simulink model "ieee80211n"  (Simulink 6.0)
settings: Solver=VariableStepDiscrete  StartTime=0.0  StopTime=inf  RelTol=1e-3
PreLoadFcn:
  | load IEEE80211n_init;
values from neighbouring files (symbols this model uses):
  params =     [IEEE80211n_init.mat]    (also in IEEE80211n_settings.m = p)
undefined symbols (not defined in the file or in its folder): magnitude
libraries: commblkintrlv2 x196, dspsigops x143, simulink x136, commdigbbndam2 x98, dspmtrx3 x96, dspsigattribs x69, dspstat3 x38, commutil2 x32, commsequence2 x26, commcnvcod2 x10, dspindex x9, dspmlti3 x8
(part 4 of 12)

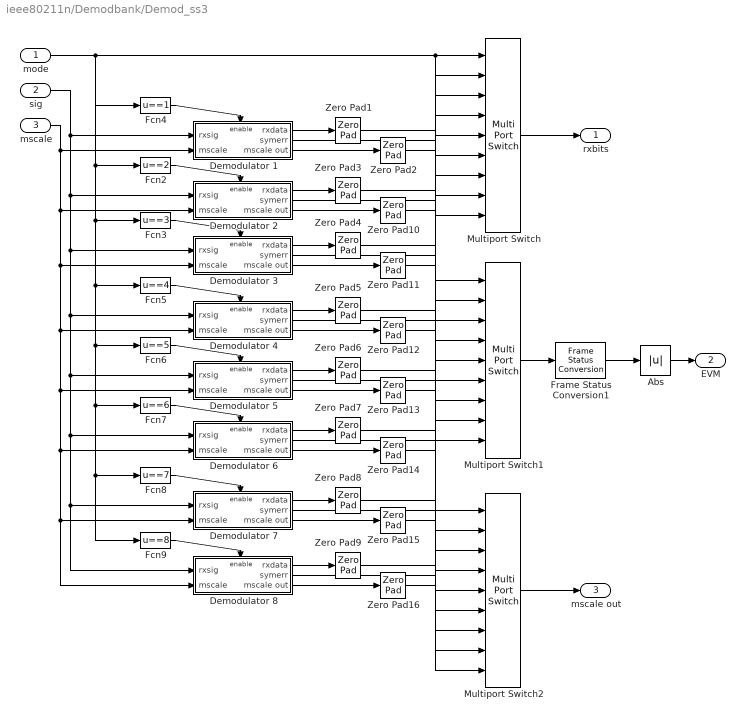
== system ieee80211n/Demodbank/Demod_ss3 ==
  mode : Inport  Port=1  LatchInput=off
  sig : Inport  Port=2  LatchInput=off
  mscale : Inport  Port=3  LatchInput=off
  Abs : Abs  SaturateOnIntegerOverflow=on
  Demodulator 1 : Subsystem  AncestorBlock=IEEE80211a_lib/Demodulator  TreatAsAtomicUnit=on  mask(QAM Demodulator-Decoder.){numSymbols=832, modulation=BPSK, code=1/2, trellisStructure=poly2trellis(7, [171 133]), punctureVector=[1], vtbd=128}
      mask prompts: numSymbols "Number of symbols per frame:"; trellisStructure "Trellis:"; punctureVector "Puncture vector:"; vtbd "Viterbi trace back depth:"
      mask help: Demodulator has option to zero-pad output, so that a bank of different modulators can share the same output frame size.
      mask init:
      | % number of bits per symbol
      | switch modulation
      | 	case 'BPSK', Nb1 = 1;
      | 	case 'QPSK', Nb1 = 2;
      | 	case '16-QAM', Nb1 = 4;
      | 	case '64-QAM', Nb1 = 6;
      | end
      | 
      | modOrder = 2.^Nb1;
      | Nb = numSymbols * Nb1; % tx bits per block
      | codeRate = str2num(strvcat(code)).';
      | bitsPerBlock = Nb .* codeRate;
      | s=max([Nb1/2 1]);
      | 
      | % interleaver
      | interleaverRows = 13;
      | if rem(Nb, interleaverRows)
      | 	error('Number of transmitted bits per block must be multiple of 16.')
      | end
      | interleaverCols = Nb / interleaverRows;
      | interleaverElements = [...
      |             s*floor( [0:Nb-1]/s ) + ...
      |             mod( ([0:Nb-1] + Nb - floor( interleaverRows*[0:Nb-1]/Nb ) ), s ) ...
      |             + 1]';
      | 	
      | if 1 %%%%%%%%%%%%%%%%%%%%%%%%
      | % freq rotation interleaver
      | iss = 2;
      | freqRotNum = 1*11;  % 20MHz channel
      | freqRotInterleaverElements = [...
      |             mod([0:Nb-1] - (mod(2*iss, 3) + 3*floor(iss/3)*freqRotNum*Nb1), Nb) ...
      |             + 1]';
      | end   %%%%%%%%%%%%%%%%%%%%%%%%
      mask Display:
      | disp(['Demodulator\n' modulation ' ' code])
      | port_label('input', 1, ' ')
      | port_label('output', 1, ' ')
      | port_label('output', 2, 'err')
  Demodulator 2 : Subsystem  AncestorBlock=IEEE80211a_lib/Demodulator  TreatAsAtomicUnit=on  mask(QAM Demodulator-Decoder.){numSymbols=832, modulation=QPSK, code=1/2, trellisStructure=poly2trellis(7, [171 133]), punctureVector=[1], vtbd=128}
      mask prompts: numSymbols "Number of symbols per frame:"; trellisStructure "Trellis:"; punctureVector "Puncture vector:"; vtbd "Viterbi trace back depth:"
      mask help: Demodulator has option to zero-pad output, so that a bank of different modulators can share the same output frame size.
      mask init: same as ieee80211n/Demodbank/Demod_ss3/Demodulator 1
      mask Display:
      | disp(['Demodulator\n' modulation ' ' code])
      | port_label('input', 1, ' ')
      | port_label('output', 1, ' ')
      | port_label('output', 2, 'err')
  Demodulator 3 : Subsystem  AncestorBlock=IEEE80211a_lib/Demodulator  TreatAsAtomicUnit=on  mask(QAM Demodulator-Decoder.){numSymbols=832, modulation=QPSK, code=3/4, trellisStructure=poly2trellis(7, [171 133]), punctureVector=[1 1 1 0 0 1].', vtbd=128}
      mask prompts: numSymbols "Number of symbols per frame:"; trellisStructure "Trellis:"; punctureVector "Puncture vector:"; vtbd "Viterbi trace back depth:"
      mask help: Demodulator has option to zero-pad output, so that a bank of different modulators can share the same output frame size.
      mask init: same as ieee80211n/Demodbank/Demod_ss3/Demodulator 1
      mask Display:
      | disp(['Demodulator\n' modulation ' ' code])
      | port_label('input', 1, ' ')
      | port_label('output', 1, ' ')
      | port_label('output', 2, 'err')
  Demodulator 4 : Subsystem  AncestorBlock=IEEE80211a_lib/Demodulator  TreatAsAtomicUnit=on  mask(QAM Demodulator-Decoder.){numSymbols=832, modulation=16-QAM, code=1/2, trellisStructure=poly2trellis(7, [171 133]), punctureVector=[1], vtbd=128}
      mask prompts: numSymbols "Number of symbols per frame:"; trellisStructure "Trellis:"; punctureVector "Puncture vector:"; vtbd "Viterbi trace back depth:"
      mask help: Demodulator has option to zero-pad output, so that a bank of different modulators can share the same output frame size.
      mask init: same as ieee80211n/Demodbank/Demod_ss3/Demodulator 1
      mask Display:
      | disp(['Demodulator\n' modulation ' ' code])
      | port_label('input', 1, ' ')
      | port_label('output', 1, ' ')
      | port_label('output', 2, 'err')
  Demodulator 5 : Subsystem  AncestorBlock=IEEE80211a_lib/Demodulator  TreatAsAtomicUnit=on  mask(QAM Demodulator-Decoder.){numSymbols=832, modulation=16-QAM, code=3/4, trellisStructure=poly2trellis(7, [171 133]), punctureVector=[1 1 1 0 0 1].', vtbd=128}
      mask prompts: numSymbols "Number of symbols per frame:"; trellisStructure "Trellis:"; punctureVector "Puncture vector:"; vtbd "Viterbi trace back depth:"
      mask help: Demodulator has option to zero-pad output, so that a bank of different modulators can share the same output frame size.
      mask init: same as ieee80211n/Demodbank/Demod_ss3/Demodulator 1
      mask Display:
      | disp(['Demodulator\n' modulation ' ' code])
      | port_label('input', 1, ' ')
      | port_label('output', 1, ' ')
      | port_label('output', 2, 'err')
  Demodulator 6 : Subsystem  AncestorBlock=IEEE80211a_lib/Demodulator  TreatAsAtomicUnit=on  mask(QAM Demodulator-Decoder.){numSymbols=832, modulation=64-QAM, code=2/3, trellisStructure=poly2trellis(7, [133 171]), punctureVector=[1 1 1 0].', vtbd=128}
      mask prompts: numSymbols "Number of symbols per frame:"; trellisStructure "Trellis:"; punctureVector "Puncture vector:"; vtbd "Viterbi trace back depth:"
      mask help: Demodulator has option to zero-pad output, so that a bank of different modulators can share the same output frame size.
      mask init: same as ieee80211n/Demodbank/Demod_ss3/Demodulator 1
      mask Display:
      | disp(['Demodulator\n' modulation ' ' code])
      | port_label('input', 1, ' ')
      | port_label('output', 1, ' ')
      | port_label('output', 2, 'err')
  Demodulator 7 : Subsystem  AncestorBlock=IEEE80211a_lib/Demodulator  TreatAsAtomicUnit=on  mask(QAM Demodulator-Decoder.){numSymbols=832, modulation=64-QAM, code=3/4, trellisStructure=poly2trellis(7, [133 171]), punctureVector=[1 1 1 0 0 1].', vtbd=128}
      mask prompts: numSymbols "Number of symbols per frame:"; trellisStructure "Trellis:"; punctureVector "Puncture vector:"; vtbd "Viterbi trace back depth:"
      mask help: Demodulator has option to zero-pad output, so that a bank of different modulators can share the same output frame size.
      mask init: same as ieee80211n/Demodbank/Demod_ss3/Demodulator 1
      mask Display:
      | disp(['Demodulator\n' modulation ' ' code])
      | port_label('input', 1, ' ')
      | port_label('output', 1, ' ')
      | port_label('output', 2, 'err')
  Demodulator 8 : Subsystem  AncestorBlock=IEEE80211a_lib/Demodulator  TreatAsAtomicUnit=on  mask(QAM Demodulator-Decoder.){numSymbols=832, modulation=64-QAM, code=5/6, trellisStructure=poly2trellis(7, [133 171]), punctureVector=[1 1 1 0 0 1 1 0 0 1].', vtbd=128}
      mask prompts: numSymbols "Number of symbols per frame:"; trellisStructure "Trellis:"; punctureVector "Puncture vector:"; vtbd "Viterbi trace back depth:"
      mask help: Demodulator has option to zero-pad output, so that a bank of different modulators can share the same output frame size.
      mask init: same as ieee80211n/Demodbank/Demod_ss3/Demodulator 1
      mask Display:
      | disp(['Demodulator\n' modulation ' ' code])
      | port_label('input', 1, ' ')
      | port_label('output', 1, ' ')
      | port_label('output', 2, 'err')
  Fcn2 : Fcn  Expr=u==2
  Fcn3 : Fcn  Expr=u==3
  Fcn4 : Fcn  Expr=u==1
  Fcn5 : Fcn  Expr=u==4
  Fcn6 : Fcn  Expr=u==5
  Fcn7 : Fcn  Expr=u==6
  Fcn8 : Fcn  Expr=u==7
  Fcn9 : Fcn  Expr=u==8
  Frame Status Conversion1 : dspsigattribs/Frame Status Conversion  growRefPort=off  outframe=Sample-based
  Multiport Switch : MultiPortSwitch  Inputs=8  SaturateOnIntegerOverflow=on
  Multiport Switch1 : MultiPortSwitch  Inputs=8  SaturateOnIntegerOverflow=on
  Multiport Switch2 : MultiPortSwitch  Inputs=8  SaturateOnIntegerOverflow=on
  Zero Pad{1..16} (16 alike) : dspsigops/Zero Pad  padSigAt=End  zpadAlong=Columns  padNumOutRowsSpecMethod=User-specified  numOutRows=params.maxTxBitsPerBlock  padNumOutColsSpecMethod=User-specified  numOutCols=1  trunc_flag=None
      settings: AttributesFormatString=\n
  rxbits : Outport
  EVM : Outport  Port=2
  mscale out : Outport  Port=3
  wires:
  sig/1 -> Demodulator 1/1(rxsig), Demodulator 3/1(rxsig), Demodulator 6/1(rxsig), Demodulator 7/1(rxsig), Demodulator 8/1(rxsig), Demodulator 5/1(rxsig), Demodulator 4/1(rxsig), Demodulator 2/1(rxsig)
  mode/1 -> Multiport Switch1/1, Multiport Switch/1, Multiport Switch2/1, Fcn4/1, Fcn7/1, Fcn8/1, Fcn9/1, Fcn6/1, Fcn5/1, Fcn3/1, Fcn2/1
  Multiport Switch/1 -> rxbits/1
  Zero Pad1/1 -> Multiport Switch/2
  Demodulator 7/1(rxdata) -> Zero Pad8/1
  Demodulator 6/1(rxdata) -> Zero Pad7/1
  Demodulator 5/1(rxdata) -> Zero Pad6/1
  Demodulator 3/1(rxdata) -> Zero Pad4/1
  Demodulator 4/1(rxdata) -> Zero Pad5/1
  Multiport Switch1/1 -> Frame Status Conversion1/1
  Demodulator 1/2(symerr) -> Multiport Switch1/2
  Demodulator 2/2(symerr) -> Multiport Switch1/3
  Demodulator 4/2(symerr) -> Multiport Switch1/5
  Demodulator 5/2(symerr) -> Multiport Switch1/6
  Demodulator 6/2(symerr) -> Multiport Switch1/7
  Demodulator 7/2(symerr) -> Multiport Switch1/8
  Demodulator 3/2(symerr) -> Multiport Switch1/4
  Zero Pad3/1 -> Multiport Switch/3
  Zero Pad4/1 -> Multiport Switch/4
  Zero Pad5/1 -> Multiport Switch/5
  Zero Pad6/1 -> Multiport Switch/6
  Zero Pad7/1 -> Multiport Switch/7
  Zero Pad8/1 -> Multiport Switch/8
  Fcn4/1 -> Demodulator 1/Enable
  Fcn2/1 -> Demodulator 2/Enable
  Fcn3/1 -> Demodulator 3/Enable
  Fcn5/1 -> Demodulator 4/Enable
  Fcn6/1 -> Demodulator 5/Enable
  Fcn7/1 -> Demodulator 6/Enable
  Fcn8/1 -> Demodulator 7/Enable
  Demodulator 1/1(rxdata) -> Zero Pad1/1
  Demodulator 2/1(rxdata) -> Zero Pad3/1
  Frame Status Conversion1/1 -> Abs/1
  Abs/1 -> EVM/1
  Demodulator 8/1(rxdata) -> Zero Pad9/1
  Demodulator 8/2(symerr) -> Multiport Switch1/9
  Zero Pad9/1 -> Multiport Switch/9
  Fcn9/1 -> Demodulator 8/Enable
  mscale/1 -> Demodulator 1/2(mscale), Demodulator 2/2(mscale), Demodulator 3/2(mscale), Demodulator 4/2(mscale), Demodulator 5/2(mscale), Demodulator 6/2(mscale), Demodulator 7/2(mscale), Demodulator 8/2(mscale)
  Multiport Switch2/1 -> mscale out/1
  Demodulator 1/3(mscale out) -> Zero Pad2/1
  Demodulator 2/3(mscale out) -> Zero Pad10/1
  Demodulator 3/3(mscale out) -> Zero Pad11/1
  Demodulator 4/3(mscale out) -> Zero Pad12/1
  Demodulator 5/3(mscale out) -> Zero Pad13/1
  Demodulator 6/3(mscale out) -> Zero Pad14/1
  Demodulator 7/3(mscale out) -> Zero Pad15/1
  Demodulator 8/3(mscale out) -> Zero Pad16/1
  Zero Pad2/1 -> Multiport Switch2/2
  Zero Pad10/1 -> Multiport Switch2/3
  Zero Pad11/1 -> Multiport Switch2/4
  Zero Pad12/1 -> Multiport Switch2/5
  Zero Pad13/1 -> Multiport Switch2/6
  Zero Pad14/1 -> Multiport Switch2/7
  Zero Pad15/1 -> Multiport Switch2/8
  Zero Pad16/1 -> Multiport Switch2/9

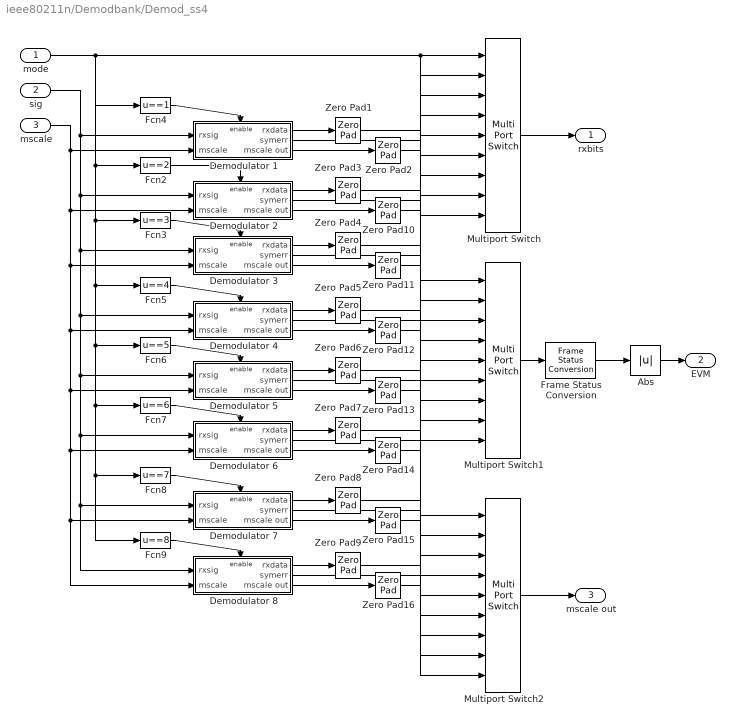
== system ieee80211n/Demodbank/Demod_ss4 ==
  mode : Inport  Port=1  LatchInput=off
  sig : Inport  Port=2  LatchInput=off
  mscale : Inport  Port=3  LatchInput=off
  Abs : Abs  SaturateOnIntegerOverflow=on
  Demodulator 1 : Subsystem  AncestorBlock=IEEE80211a_lib/Demodulator  TreatAsAtomicUnit=on  mask(QAM Demodulator-Decoder.){numSymbols=832, modulation=BPSK, code=1/2, trellisStructure=poly2trellis(7, [171 133]), punctureVector=[1], vtbd=128}
      mask prompts: numSymbols "Number of symbols per frame:"; trellisStructure "Trellis:"; punctureVector "Puncture vector:"; vtbd "Viterbi trace back depth:"
      mask help: Demodulator has option to zero-pad output, so that a bank of different modulators can share the same output frame size.
      mask init:
      | % number of bits per symbol
      | switch modulation
      | 	case 'BPSK', Nb1 = 1;
      | 	case 'QPSK', Nb1 = 2;
      | 	case '16-QAM', Nb1 = 4;
      | 	case '64-QAM', Nb1 = 6;
      | end
      | 
      | modOrder = 2.^Nb1;
      | Nb = numSymbols * Nb1; % tx bits per block
      | codeRate = str2num(strvcat(code)).';
      | bitsPerBlock = Nb .* codeRate;
      | s=max([Nb1/2 1]);
      | 
      | % interleaver
      | interleaverRows = 13;
      | if rem(Nb, interleaverRows)
      | 	error('Number of transmitted bits per block must be multiple of 16.')
      | end
      | interleaverCols = Nb / interleaverRows;
      | interleaverElements = [...
      |             s*floor( [0:Nb-1]/s ) + ...
      |             mod( ([0:Nb-1] + Nb - floor( interleaverRows*[0:Nb-1]/Nb ) ), s ) ...
      |             + 1]';
      | 	
      | if 1 %%%%%%%%%%%%%%%%%%%%%%%%
      | % freq rotation interleaver
      | iss = 3;
      | freqRotNum = 3*11;  % 20MHz channel
      | freqRotInterleaverElements = [...
      |             mod([0:Nb-1] - (mod(2*iss, 3) + 3*floor(iss/3)*freqRotNum*Nb1), Nb) ...
      |             + 1]';
      | end   %%%%%%%%%%%%%%%%%%%%%%%%
      mask Display:
      | disp(['Demodulator\n' modulation ' ' code])
      | port_label('input', 1, ' ')
      | port_label('output', 1, ' ')
      | port_label('output', 2, 'err')
  Demodulator 2 : Subsystem  AncestorBlock=IEEE80211a_lib/Demodulator  TreatAsAtomicUnit=on  mask(QAM Demodulator-Decoder.){numSymbols=832, modulation=QPSK, code=1/2, trellisStructure=poly2trellis(7, [171 133]), punctureVector=[1], vtbd=128}
      mask prompts: numSymbols "Number of symbols per frame:"; trellisStructure "Trellis:"; punctureVector "Puncture vector:"; vtbd "Viterbi trace back depth:"
      mask help: Demodulator has option to zero-pad output, so that a bank of different modulators can share the same output frame size.
      mask init: same as ieee80211n/Demodbank/Demod_ss4/Demodulator 1
      mask Display:
      | disp(['Demodulator\n' modulation ' ' code])
      | port_label('input', 1, ' ')
      | port_label('output', 1, ' ')
      | port_label('output', 2, 'err')
  Demodulator 3 : Subsystem  AncestorBlock=IEEE80211a_lib/Demodulator  TreatAsAtomicUnit=on  mask(QAM Demodulator-Decoder.){numSymbols=832, modulation=QPSK, code=3/4, trellisStructure=poly2trellis(7, [171 133]), punctureVector=[1 1 1 0 0 1].', vtbd=128}
      mask prompts: numSymbols "Number of symbols per frame:"; trellisStructure "Trellis:"; punctureVector "Puncture vector:"; vtbd "Viterbi trace back depth:"
      mask help: Demodulator has option to zero-pad output, so that a bank of different modulators can share the same output frame size.
      mask init: same as ieee80211n/Demodbank/Demod_ss4/Demodulator 1
      mask Display:
      | disp(['Demodulator\n' modulation ' ' code])
      | port_label('input', 1, ' ')
      | port_label('output', 1, ' ')
      | port_label('output', 2, 'err')
  Demodulator 4 : Subsystem  AncestorBlock=IEEE80211a_lib/Demodulator  TreatAsAtomicUnit=on  mask(QAM Demodulator-Decoder.){numSymbols=832, modulation=16-QAM, code=1/2, trellisStructure=poly2trellis(7, [171 133]), punctureVector=[1], vtbd=128}
      mask prompts: numSymbols "Number of symbols per frame:"; trellisStructure "Trellis:"; punctureVector "Puncture vector:"; vtbd "Viterbi trace back depth:"
      mask help: Demodulator has option to zero-pad output, so that a bank of different modulators can share the same output frame size.
      mask init: same as ieee80211n/Demodbank/Demod_ss4/Demodulator 1
      mask Display:
      | disp(['Demodulator\n' modulation ' ' code])
      | port_label('input', 1, ' ')
      | port_label('output', 1, ' ')
      | port_label('output', 2, 'err')
  Demodulator 5 : Subsystem  AncestorBlock=IEEE80211a_lib/Demodulator  TreatAsAtomicUnit=on  mask(QAM Demodulator-Decoder.){numSymbols=832, modulation=16-QAM, code=3/4, trellisStructure=poly2trellis(7, [171 133]), punctureVector=[1 1 1 0 0 1].', vtbd=128}
      mask prompts: numSymbols "Number of symbols per frame:"; trellisStructure "Trellis:"; punctureVector "Puncture vector:"; vtbd "Viterbi trace back depth:"
      mask help: Demodulator has option to zero-pad output, so that a bank of different modulators can share the same output frame size.
      mask init: same as ieee80211n/Demodbank/Demod_ss4/Demodulator 1
      mask Display:
      | disp(['Demodulator\n' modulation ' ' code])
      | port_label('input', 1, ' ')
      | port_label('output', 1, ' ')
      | port_label('output', 2, 'err')
  Demodulator 6 : Subsystem  AncestorBlock=IEEE80211a_lib/Demodulator  TreatAsAtomicUnit=on  mask(QAM Demodulator-Decoder.){numSymbols=832, modulation=64-QAM, code=2/3, trellisStructure=poly2trellis(7, [133 171]), punctureVector=[1 1 1 0].', vtbd=128}
      mask prompts: numSymbols "Number of symbols per frame:"; trellisStructure "Trellis:"; punctureVector "Puncture vector:"; vtbd "Viterbi trace back depth:"
      mask help: Demodulator has option to zero-pad output, so that a bank of different modulators can share the same output frame size.
      mask init: same as ieee80211n/Demodbank/Demod_ss4/Demodulator 1
      mask Display:
      | disp(['Demodulator\n' modulation ' ' code])
      | port_label('input', 1, ' ')
      | port_label('output', 1, ' ')
      | port_label('output', 2, 'err')
  Demodulator 7 : Subsystem  AncestorBlock=IEEE80211a_lib/Demodulator  TreatAsAtomicUnit=on  mask(QAM Demodulator-Decoder.){numSymbols=832, modulation=64-QAM, code=3/4, trellisStructure=poly2trellis(7, [133 171]), punctureVector=[1 1 1 0 0 1].', vtbd=128}
      mask prompts: numSymbols "Number of symbols per frame:"; trellisStructure "Trellis:"; punctureVector "Puncture vector:"; vtbd "Viterbi trace back depth:"
      mask help: Demodulator has option to zero-pad output, so that a bank of different modulators can share the same output frame size.
      mask init: same as ieee80211n/Demodbank/Demod_ss4/Demodulator 1
      mask Display:
      | disp(['Demodulator\n' modulation ' ' code])
      | port_label('input', 1, ' ')
      | port_label('output', 1, ' ')
      | port_label('output', 2, 'err')
  Demodulator 8 : Subsystem  AncestorBlock=IEEE80211a_lib/Demodulator  TreatAsAtomicUnit=on  mask(QAM Demodulator-Decoder.){numSymbols=832, modulation=64-QAM, code=5/6, trellisStructure=poly2trellis(7, [133 171]), punctureVector=[1 1 1 0 0 1 1 0 0 1].', vtbd=128}
      mask prompts: numSymbols "Number of symbols per frame:"; trellisStructure "Trellis:"; punctureVector "Puncture vector:"; vtbd "Viterbi trace back depth:"
      mask help: Demodulator has option to zero-pad output, so that a bank of different modulators can share the same output frame size.
      mask init: same as ieee80211n/Demodbank/Demod_ss4/Demodulator 1
      mask Display:
      | disp(['Demodulator\n' modulation ' ' code])
      | port_label('input', 1, ' ')
      | port_label('output', 1, ' ')
      | port_label('output', 2, 'err')
  Fcn2 : Fcn  Expr=u==2
  Fcn3 : Fcn  Expr=u==3
  Fcn4 : Fcn  Expr=u==1
  Fcn5 : Fcn  Expr=u==4
  Fcn6 : Fcn  Expr=u==5
  Fcn7 : Fcn  Expr=u==6
  Fcn8 : Fcn  Expr=u==7
  Fcn9 : Fcn  Expr=u==8
  Frame Status Conversion : dspsigattribs/Frame Status Conversion  growRefPort=off  outframe=Sample-based
  Multiport Switch : MultiPortSwitch  Inputs=8  SaturateOnIntegerOverflow=on
  Multiport Switch1 : MultiPortSwitch  Inputs=8  SaturateOnIntegerOverflow=on
  Multiport Switch2 : MultiPortSwitch  Inputs=8  SaturateOnIntegerOverflow=on
  Zero Pad{1..16} (16 alike) : dspsigops/Zero Pad  padSigAt=End  zpadAlong=Columns  padNumOutRowsSpecMethod=User-specified  numOutRows=params.maxTxBitsPerBlock  padNumOutColsSpecMethod=User-specified  numOutCols=1  trunc_flag=None
      settings: AttributesFormatString=\n
  rxbits : Outport
  EVM : Outport  Port=2
  mscale out : Outport  Port=3
  wires:
  sig/1 -> Demodulator 1/1(rxsig), Demodulator 3/1(rxsig), Demodulator 6/1(rxsig), Demodulator 7/1(rxsig), Demodulator 8/1(rxsig), Demodulator 5/1(rxsig), Demodulator 4/1(rxsig), Demodulator 2/1(rxsig)
  mode/1 -> Multiport Switch1/1, Multiport Switch/1, Multiport Switch2/1, Fcn4/1, Fcn7/1, Fcn8/1, Fcn9/1, Fcn6/1, Fcn5/1, Fcn3/1, Fcn2/1
  Multiport Switch/1 -> rxbits/1
  Zero Pad1/1 -> Multiport Switch/2
  Demodulator 7/1(rxdata) -> Zero Pad8/1
  Demodulator 6/1(rxdata) -> Zero Pad7/1
  Demodulator 5/1(rxdata) -> Zero Pad6/1
  Demodulator 3/1(rxdata) -> Zero Pad4/1
  Demodulator 4/1(rxdata) -> Zero Pad5/1
  Multiport Switch1/1 -> Frame Status Conversion/1
  Demodulator 1/2(symerr) -> Multiport Switch1/2
  Demodulator 2/2(symerr) -> Multiport Switch1/3
  Demodulator 4/2(symerr) -> Multiport Switch1/5
  Demodulator 5/2(symerr) -> Multiport Switch1/6
  Demodulator 6/2(symerr) -> Multiport Switch1/7
  Demodulator 7/2(symerr) -> Multiport Switch1/8
  Demodulator 3/2(symerr) -> Multiport Switch1/4
  Zero Pad3/1 -> Multiport Switch/3
  Zero Pad4/1 -> Multiport Switch/4
  Zero Pad5/1 -> Multiport Switch/5
  Zero Pad6/1 -> Multiport Switch/6
  Zero Pad7/1 -> Multiport Switch/7
  Zero Pad8/1 -> Multiport Switch/8
  Fcn4/1 -> Demodulator 1/Enable
  Fcn2/1 -> Demodulator 2/Enable
  Fcn3/1 -> Demodulator 3/Enable
  Fcn5/1 -> Demodulator 4/Enable
  Fcn6/1 -> Demodulator 5/Enable
  Fcn7/1 -> Demodulator 6/Enable
  Fcn8/1 -> Demodulator 7/Enable
  Demodulator 1/1(rxdata) -> Zero Pad1/1
  Demodulator 2/1(rxdata) -> Zero Pad3/1
  Frame Status Conversion/1 -> Abs/1
  Abs/1 -> EVM/1
  Demodulator 8/1(rxdata) -> Zero Pad9/1
  Demodulator 8/2(symerr) -> Multiport Switch1/9
  Zero Pad9/1 -> Multiport Switch/9
  Fcn9/1 -> Demodulator 8/Enable
  mscale/1 -> Demodulator 1/2(mscale), Demodulator 2/2(mscale), Demodulator 3/2(mscale), Demodulator 4/2(mscale), Demodulator 5/2(mscale), Demodulator 6/2(mscale), Demodulator 7/2(mscale), Demodulator 8/2(mscale)
  Multiport Switch2/1 -> mscale out/1
  Demodulator 1/3(mscale out) -> Zero Pad2/1
  Demodulator 2/3(mscale out) -> Zero Pad10/1
  Demodulator 3/3(mscale out) -> Zero Pad11/1
  Demodulator 4/3(mscale out) -> Zero Pad12/1
  Demodulator 5/3(mscale out) -> Zero Pad13/1
  Demodulator 6/3(mscale out) -> Zero Pad14/1
  Demodulator 7/3(mscale out) -> Zero Pad15/1
  Demodulator 8/3(mscale out) -> Zero Pad16/1
  Zero Pad2/1 -> Multiport Switch2/2
  Zero Pad10/1 -> Multiport Switch2/3
  Zero Pad11/1 -> Multiport Switch2/4
  Zero Pad12/1 -> Multiport Switch2/5
  Zero Pad13/1 -> Multiport Switch2/6
  Zero Pad14/1 -> Multiport Switch2/7
  Zero Pad15/1 -> Multiport Switch2/8
  Zero Pad16/1 -> Multiport Switch2/9

== system ieee80211n/DocBlock/EmptySubsystem ==

== system ieee80211n/MATLAB graphics/Transform data ==
  in : Inport  Port=1  LatchInput=off
  Complex to Real-Imag : ComplexToRealImag
  Concatenate : simulink/Math Operations/Matrix Concatenation  numInports=2  catMethod=Horizontal
  Frame Status Conversion1 : dspsigattribs/Frame Status Conversion  growRefPort=off  outframe=Sample-based
  out : Outport
  wires:
  Frame Status Conversion1/1 -> out/1
  in/1 -> Complex to Real-Imag/1
  Complex to Real-Imag/1 -> Concatenate/1
  Complex to Real-Imag/2 -> Concatenate/2
  Concatenate/1 -> Frame Status Conversion1/1

== system ieee80211n/MATLAB graphics/append1 ==
  in : Inport  Port=1  LatchInput=off
  Matrix Concatenation1 : simulink/Math Operations/Matrix Concatenation  numInports=2  catMethod=Vertical
  Reshape : simulink/Math Operations/Reshape  OutputDimensionality=Column vector  OutputDimensions=[1,1]
  Transpose : dspmtrx3/Transpose  Hermitian=off  overflowFlag=on
      settings: AttributesFormatString=\n
  Width : Width
  out : Outport
  wires:
  in/1 -> Width/1, Reshape/1
  Width/1 -> Transpose/1
  Reshape/1 -> Matrix Concatenation1/2
  Transpose/1 -> Matrix Concatenation1/1
  Matrix Concatenation1/1 -> out/1

== system ieee80211n/MATLAB graphics/append2 ==
  in : Inport  Port=1  LatchInput=off
  Matrix Concatenation1 : simulink/Math Operations/Matrix Concatenation  numInports=2  catMethod=Vertical
  Reshape : simulink/Math Operations/Reshape  OutputDimensionality=Column vector  OutputDimensions=[1,1]
  Transpose : dspmtrx3/Transpose  Hermitian=off  overflowFlag=on
      settings: AttributesFormatString=\n
  Width : Width
  out : Outport
  wires:
  Matrix Concatenation1/1 -> out/1
  Transpose/1 -> Matrix Concatenation1/1
  Reshape/1 -> Matrix Concatenation1/2
  Width/1 -> Transpose/1
  in/1 -> Reshape/1, Width/1

== system ieee80211n/MATLAB graphics/append3 ==
  in : Inport  Port=1  LatchInput=off
  Matrix Concatenation1 : simulink/Math Operations/Matrix Concatenation  numInports=2  catMethod=Vertical
  Reshape : simulink/Math Operations/Reshape  OutputDimensionality=Column vector  OutputDimensions=[1,1]
  Transpose : dspmtrx3/Transpose  Hermitian=off  overflowFlag=on
      settings: AttributesFormatString=\n
  Width : Width
  out : Outport
  wires:
  Matrix Concatenation1/1 -> out/1
  Transpose/1 -> Matrix Concatenation1/1
  Reshape/1 -> Matrix Concatenation1/2
  Width/1 -> Transpose/1
  in/1 -> Reshape/1, Width/1

== system ieee80211n/MATLAB graphics/append5 ==
  in : Inport  Port=1  LatchInput=off
  Matrix Concatenation1 : simulink/Math Operations/Matrix Concatenation  numInports=2  catMethod=Vertical
  Reshape : simulink/Math Operations/Reshape  OutputDimensionality=Column vector  OutputDimensions=[1,1]
  Transpose : dspmtrx3/Transpose  Hermitian=off  overflowFlag=on
      settings: AttributesFormatString=\n
  Width : Width
  out : Outport
  wires:
  Matrix Concatenation1/1 -> out/1
  Transpose/1 -> Matrix Concatenation1/1
  Reshape/1 -> Matrix Concatenation1/2
  Width/1 -> Transpose/1
  in/1 -> Reshape/1, Width/1

== system ieee80211n/MATLAB graphics/append6 ==
  in : Inport  Port=1  LatchInput=off
  Matrix Concatenation1 : simulink/Math Operations/Matrix Concatenation  numInports=2  catMethod=Vertical
  Reshape : simulink/Math Operations/Reshape  OutputDimensionality=Column vector  OutputDimensions=[1,1]
  Transpose : dspmtrx3/Transpose  Hermitian=off  overflowFlag=on
      settings: AttributesFormatString=\n
  Width : Width
  out : Outport
  wires:
  Matrix Concatenation1/1 -> out/1
  Transpose/1 -> Matrix Concatenation1/1
  Reshape/1 -> Matrix Concatenation1/2
  Width/1 -> Transpose/1
  in/1 -> Reshape/1, Width/1

== system ieee80211n/MATLAB graphics/append7 ==
  in : Inport  Port=1  LatchInput=off
  Matrix Concatenation1 : simulink/Math Operations/Matrix Concatenation  numInports=2  catMethod=Vertical
  Reshape : simulink/Math Operations/Reshape  OutputDimensionality=Column vector  OutputDimensions=[1,1]
  Transpose : dspmtrx3/Transpose  Hermitian=off  overflowFlag=on
      settings: AttributesFormatString=\n
  Width : Width
  out : Outport
  wires:
  Matrix Concatenation1/1 -> out/1
  Transpose/1 -> Matrix Concatenation1/1
  Reshape/1 -> Matrix Concatenation1/2
  Width/1 -> Transpose/1
  in/1 -> Reshape/1, Width/1

== system ieee80211n/MATLAB graphics/append8 ==
  in : Inport  Port=1  LatchInput=off
  Matrix Concatenation1 : simulink/Math Operations/Matrix Concatenation  numInports=2  catMethod=Vertical
  Reshape : simulink/Math Operations/Reshape  OutputDimensionality=Column vector  OutputDimensions=[1,1]
  Transpose : dspmtrx3/Transpose  Hermitian=off  overflowFlag=on
      settings: AttributesFormatString=\n
  Width : Width
  out : Outport
  wires:
  Matrix Concatenation1/1 -> out/1
  Transpose/1 -> Matrix Concatenation1/1
  Reshape/1 -> Matrix Concatenation1/2
  Width/1 -> Transpose/1
  in/1 -> Reshape/1, Width/1

== system ieee80211n/MATLAB graphics/append9 ==
  in : Inport  Port=1  LatchInput=off
  Matrix Concatenation1 : simulink/Math Operations/Matrix Concatenation  numInports=2  catMethod=Vertical
  Reshape : simulink/Math Operations/Reshape  OutputDimensionality=Column vector  OutputDimensions=[1,1]
  Transpose : dspmtrx3/Transpose  Hermitian=off  overflowFlag=on
      settings: AttributesFormatString=\n
  Width : Width
  out : Outport
  wires:
  Matrix Concatenation1/1 -> out/1
  Transpose/1 -> Matrix Concatenation1/1
  Reshape/1 -> Matrix Concatenation1/2
  Width/1 -> Transpose/1
  in/1 -> Reshape/1, Width/1

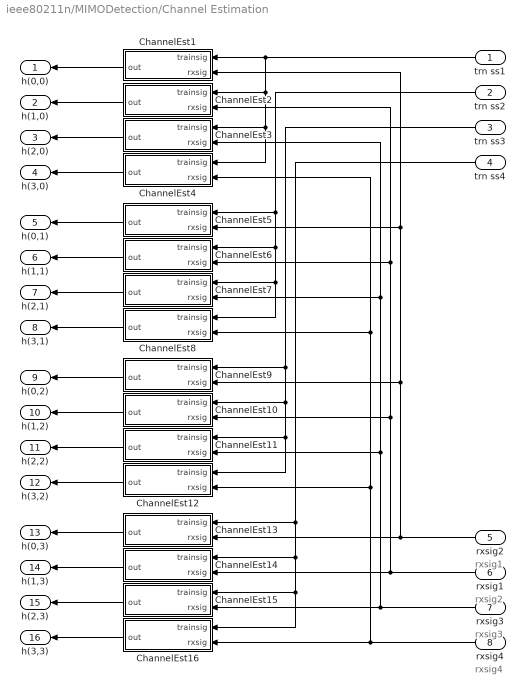
== system ieee80211n/MIMODetection/Channel Estimation ==
  note: rxsig1
  note: rxsig2
  note: rxsig3
  note: rxsig4
  trn ss1 : Inport  Orientation=left  Port=1  LatchInput=off
  trn ss2 : Inport  Orientation=left  Port=2  LatchInput=off
  trn ss3 : Inport  Orientation=left  Port=3  LatchInput=off
  trn ss4 : Inport  Orientation=left  Port=4  LatchInput=off
  rxsig2 : Inport  Orientation=left  Port=5  LatchInput=off
  rxsig1 : Inport  Orientation=left  Port=6  LatchInput=off
  rxsig3 : Inport  Orientation=left  Port=7  LatchInput=off
  rxsig4 : Inport  Orientation=left  Port=8  LatchInput=off
  ChannelEst1 : Subsystem  Orientation=left
      mask Display: disp('Channel Est.\nH(0,0)')
  ChannelEst10 : Subsystem  Orientation=left
      mask Display: disp('Channel Est.\nH(1,2)')
  ChannelEst11 : Subsystem  Orientation=left
      mask Display: disp('Channel Est.\nH(2,2)')
  ChannelEst12 : Subsystem  Orientation=left
      mask Display: disp('Channel Est.\nH(3,2)')
  ChannelEst13 : Subsystem  Orientation=left
      mask Display: disp('Channel Est.\nH(0,3)')
  ChannelEst14 : Subsystem  Orientation=left
      mask Display: disp('Channel Est.\nH(1,3)')
  ChannelEst15 : Subsystem  Orientation=left
      mask Display: disp('Channel Est.\nH(2,3)')
  ChannelEst16 : Subsystem  Orientation=left
      mask Display: disp('Channel Est.\nH(3,3)')
  ChannelEst2 : Subsystem  Orientation=left
      mask Display: disp('Channel Est.\nH(1,0)')
  ChannelEst3 : Subsystem  Orientation=left
      mask Display: disp('Channel Est.\nH(2,0)')
  ChannelEst4 : Subsystem  Orientation=left
      mask Display: disp('Channel Est.\nH(3,0)')
  ChannelEst5 : Subsystem  Orientation=left
      mask Display: disp('Channel Est.\nH(0,1)')
  ChannelEst6 : Subsystem  Orientation=left
      mask Display: disp('Channel Est.\nH(1,1)')
  ChannelEst7 : Subsystem  Orientation=left
      mask Display: disp('Channel Est.\nH(2,1)')
  ChannelEst8 : Subsystem  Orientation=left
      mask Display: disp('Channel Est.\nH(3,1)')
  ChannelEst9 : Subsystem  Orientation=left
      mask Display: disp('Channel Est.\nH(0,2)')
  h(0,0) : Outport  Orientation=left
  h(1,0) : Outport  Orientation=left  Port=2
  h(2,0) : Outport  Orientation=left  Port=3
  h(3,0) : Outport  Orientation=left  Port=4
  h(0,1) : Outport  Orientation=left  Port=5
  h(1,1) : Outport  Orientation=left  Port=6
  h(2,1) : Outport  Orientation=left  Port=7
  h(3,1) : Outport  Orientation=left  Port=8
  h(0,2) : Outport  Orientation=left  Port=9
  h(1,2) : Outport  Orientation=left  Port=10
  h(2,2) : Outport  Orientation=left  Port=11
  h(3,2) : Outport  Orientation=left  Port=12
  h(0,3) : Outport  Orientation=left  Port=13
  h(1,3) : Outport  Orientation=left  Port=14
  h(2,3) : Outport  Orientation=left  Port=15
  h(3,3) : Outport  Orientation=left  Port=16
  wires:
  trn ss1/1 -> ChannelEst3/1(trainsig), ChannelEst4/1(trainsig), ChannelEst2/1(trainsig), ChannelEst1/1(trainsig)
  trn ss2/1 -> ChannelEst7/1(trainsig), ChannelEst8/1(trainsig), ChannelEst6/1(trainsig), ChannelEst5/1(trainsig)
  trn ss3/1 -> ChannelEst11/1(trainsig), ChannelEst12/1(trainsig), ChannelEst10/1(trainsig), ChannelEst9/1(trainsig)
  trn ss4/1 -> ChannelEst15/1(trainsig), ChannelEst16/1(trainsig), ChannelEst14/1(trainsig), ChannelEst13/1(trainsig)
  rxsig4/1 -> ChannelEst4/2(rxsig), ChannelEst8/2(rxsig), ChannelEst12/2(rxsig), ChannelEst16/2(rxsig)
  rxsig3/1 -> ChannelEst3/2(rxsig), ChannelEst7/2(rxsig), ChannelEst11/2(rxsig), ChannelEst15/2(rxsig)
  rxsig1/1 -> ChannelEst2/2(rxsig), ChannelEst6/2(rxsig), ChannelEst10/2(rxsig), ChannelEst14/2(rxsig)
  rxsig2/1 -> ChannelEst1/2(rxsig), ChannelEst5/2(rxsig), ChannelEst9/2(rxsig), ChannelEst13/2(rxsig)
  ChannelEst1/1(out) -> h(0,0)/1
  ChannelEst2/1(out) -> h(1,0)/1
  ChannelEst3/1(out) -> h(2,0)/1
  ChannelEst4/1(out) -> h(3,0)/1
  ChannelEst5/1(out) -> h(0,1)/1
  ChannelEst6/1(out) -> h(1,1)/1
  ChannelEst7/1(out) -> h(2,1)/1
  ChannelEst8/1(out) -> h(3,1)/1
  ChannelEst9/1(out) -> h(0,2)/1
  ChannelEst10/1(out) -> h(1,2)/1
  ChannelEst11/1(out) -> h(2,2)/1
  ChannelEst12/1(out) -> h(3,2)/1
  ChannelEst13/1(out) -> h(0,3)/1
  ChannelEst14/1(out) -> h(1,3)/1
  ChannelEst15/1(out) -> h(2,3)/1
  ChannelEst16/1(out) -> h(3,3)/1

== system ieee80211n/ModulatorBank/CC_PuncBank ==
  mode : Inport  Port=1  LatchInput=off
  txbits : Inport  Port=2  LatchInput=off
  Fcn2 : Fcn  Expr=u==1
  Fcn3 : Fcn  Expr=u==2
  Fcn4 : Fcn  Expr=u==3
  Fcn5 : Fcn  Expr=u==4
  Fcn6 : Fcn  Expr=u==5
  Fcn7 : Fcn  Expr=u==6
  Fcn8 : Fcn  Expr=u==7
  Fcn9 : Fcn  Expr=u==8
  Merge1 : Merge  Inputs=8
  Modulator 1 : Subsystem  AncestorBlock=IEEE80211a_lib/Modulator  TreatAsAtomicUnit=on  mask(CC+Puncture){numSymbols=params.NSS*params.numTxSymbols, modulation=BPSK, code=1/2, trellisStructure=poly2trellis(7, [171 133]), punctureVector=[1]}
      mask prompts: numSymbols "Number of symbols per frame:"; trellisStructure "Trellis:"; punctureVector "Puncture vector:"
      mask help: Convolutional Coding and Puncturing
      mask init:
      | % number of bits per symbol
      | switch modulation
      | 	case 'BPSK', Nb1 = 1;
      | 	case 'QPSK', Nb1 = 2;
      | 	case '16-QAM', Nb1 = 4;
      | 	case '64-QAM', Nb1 = 6;
      | end
      | 
      | Nb_max = numSymbols * 6; % tx bits per block
      | 
      | modOrder = 2.^Nb1;
      | Nb = numSymbols * Nb1; % tx bits per block
      | codeRate = str2num(strvcat(code)).';
      | bitsPerBlock = Nb .* codeRate;
      | s=max([Nb1/2 1]);
      | 
      | % interleaver
      | interleaverRows = 13;
      | if rem(Nb, interleaverRows)
      | 	error('Number of transmitted bits per block must be multiple of 16.')
      | end
      | interleaverCols = Nb / interleaverRows;
      | interleaverElements = [...
      |             s*floor( [0:Nb-1]/s ) + ...
      |             mod( ([0:Nb-1] + Nb - floor( interleaverRows*[0:Nb-1]/Nb ) ), s ) ...
      |             + 1]';
      mask Display: disp(['CC+Puncture\n' 'Rate=' code])
  Modulator 2 : Subsystem  AncestorBlock=IEEE80211a_lib/Modulator  TreatAsAtomicUnit=on  mask(CC+Puncture){numSymbols=params.NSS*params.numTxSymbols, modulation=QPSK, code=1/2, trellisStructure=poly2trellis(7, [171 133]), punctureVector=[1]}
      mask prompts: numSymbols "Number of symbols per frame:"; trellisStructure "Trellis:"; punctureVector "Puncture vector:"
      mask help: Convolutional Coding and Puncturing
      mask init: same as ieee80211n/ModulatorBank/CC_PuncBank/Modulator 1
      mask Display: disp(['CC+Puncture\n' 'Rate=' code])
  Modulator 3 : Subsystem  AncestorBlock=IEEE80211a_lib/Modulator  TreatAsAtomicUnit=on  mask(CC+Puncture){numSymbols=params.NSS*params.numTxSymbols, modulation=QPSK, code=3/4, trellisStructure=poly2trellis(7, [171 133]), punctureVector=[1 1 1 0 0 1].'}
      mask prompts: numSymbols "Number of symbols per frame:"; trellisStructure "Trellis:"; punctureVector "Puncture vector:"
      mask help: Convolutional Coding and Puncturing
      mask init: same as ieee80211n/ModulatorBank/CC_PuncBank/Modulator 1
      mask Display: disp(['CC+Puncture\n' 'Rate=' code])
  Modulator 4 : Subsystem  AncestorBlock=IEEE80211a_lib/Modulator  TreatAsAtomicUnit=on  mask(CC+Puncture){numSymbols=params.NSS*params.numTxSymbols, modulation=16-QAM, code=1/2, trellisStructure=poly2trellis(7, [171 133]), punctureVector=[1]}
      mask prompts: numSymbols "Number of symbols per frame:"; trellisStructure "Trellis:"; punctureVector "Puncture vector:"
      mask help: Convolutional Coding and Puncturing
      mask init: same as ieee80211n/ModulatorBank/CC_PuncBank/Modulator 1
      mask Display: disp(['CC+Puncture\n' 'Rate=' code])
  Modulator 5 : Subsystem  AncestorBlock=IEEE80211a_lib/Modulator  TreatAsAtomicUnit=on  mask(CC+Puncture){numSymbols=params.NSS*params.numTxSymbols, modulation=16-QAM, code=3/4, trellisStructure=poly2trellis(7, [171 133]), punctureVector=[1 1 1 0 0 1].'}
      mask prompts: numSymbols "Number of symbols per frame:"; trellisStructure "Trellis:"; punctureVector "Puncture vector:"
      mask help: Convolutional Coding and Puncturing
      mask init:
      | % number of bits per symbol
      | switch modulation
      | 	case 'BPSK', Nb1 = 1;
      | 	case 'QPSK', Nb1 = 2;
      | 	case '16-QAM', Nb1 = 4;
      | 	case '64-QAM', Nb1 = 6;
      | end
      | 
      | Nb_max = numSymbols * 6; % tx bits per block
      | 
      | modOrder = 2.^Nb1;
      | Nb = numSymbols * Nb1; % tx bits per block
      | codeRate = str2num(strvcat(code)).';
      | bitsPerBlock = Nb .* codeRate;
      | 
      | % interleaver
      | interleaverRows = 13;
      | if rem(Nb, interleaverRows)
      | 	error('Number of transmitted bits per block must be multiple of 16.')
      | end
      | interleaverCols = Nb / interleaverRows;
      | interleaverElements = [...
      |             2*floor( [0:Nb-1]/2 ) + ...
      |             mod( ([0:Nb-1] + Nb - floor( interleaverRows*[0:Nb-1]/Nb ) ), 2 ) ...
      |             + 1]';
      mask Display: disp(['CC+Puncture\n' 'Rate=' code])
  Modulator 6 : Subsystem  AncestorBlock=IEEE80211a_lib/Modulator  TreatAsAtomicUnit=on  mask(CC+Puncture){numSymbols=params.NSS*params.numTxSymbols, modulation=64-QAM, code=2/3, trellisStructure=poly2trellis(7, [133 171]), punctureVector=[1 1 1 0].'}
      mask prompts: numSymbols "Number of symbols per frame:"; trellisStructure "Trellis:"; punctureVector "Puncture vector:"
      mask help: Convolutional Coding and Puncturing
      mask init: same as ieee80211n/ModulatorBank/CC_PuncBank/Modulator 1
      mask Display: disp(['CC+Puncture\n' 'Rate=' code])
  Modulator 7 : Subsystem  AncestorBlock=IEEE80211a_lib/Modulator  TreatAsAtomicUnit=on  mask(CC+Puncture){numSymbols=params.NSS*params.numTxSymbols, modulation=64-QAM, code=3/4, trellisStructure=poly2trellis(7, [133 171]), punctureVector=[1 1 1 0 0 1].'}
      mask prompts: numSymbols "Number of symbols per frame:"; trellisStructure "Trellis:"; punctureVector "Puncture vector:"
      mask help: Convolutional Coding and Puncturing
      mask init:
      | % number of bits per symbol
      | switch modulation
      | 	case 'BPSK', Nb1 = 1;
      | 	case 'QPSK', Nb1 = 2;
      | 	case '16-QAM', Nb1 = 4;
      | 	case '64-QAM', Nb1 = 6;
      | end
      | 
      | Nb_max = numSymbols * 6; % tx bits per block
      | 
      | modOrder = 2.^Nb1;
      | Nb = numSymbols * Nb1; % tx bits per block
      | codeRate = str2num(strvcat(code)).';
      | bitsPerBlock = Nb .* codeRate;
      | s=max([Nb1/2 1]);
      | 
      | % interleaver
      | interleaverRows = 13;
      | if rem(Nb, interleaverRows)
      | 	error('Number of transmitted bits per block must be multiple of 16.')
      | end
      | interleaverCols = Nb / interleaverRows;
      | interleaverElements = [...
      |             s*floor( [0:Nb-1]/s ) + ...
      |             mod( ([0:Nb-1] + Nb - floor( interleaverRows*[0:Nb-1]/Nb ) ), s ) ...
      |             + 1]';
      mask Display: disp(['CC+Puncture\n' 'Rate=' code])
  Modulator 8 : Subsystem  AncestorBlock=IEEE80211a_lib/Modulator  TreatAsAtomicUnit=on  mask(CC+Puncture){numSymbols=params.NSS*params.numTxSymbols, modulation=64-QAM, code=5/6, trellisStructure=poly2trellis(7, [133 171]), punctureVector=[1 1 1 0 0 1 1 0 0 1].'}
      mask prompts: numSymbols "Number of symbols per frame:"; trellisStructure "Trellis:"; punctureVector "Puncture vector:"
      mask help: Convolutional Coding and Puncturing
      mask init: same as ieee80211n/ModulatorBank/CC_PuncBank/Modulator 1
      mask Display: disp(['CC+Puncture\n' 'Rate=' code])
  sig : Outport
  wires:
  Merge1/1 -> sig/1
  mode/1 -> Fcn2/1, Fcn7/1, Fcn8/1, Fcn9/1, Fcn6/1, Fcn5/1, Fcn4/1, Fcn3/1
  txbits/1 -> Modulator 1/1(txdata), Modulator 7/1(txdata), Modulator 8/1(txdata), Modulator 6/1(txdata), Modulator 5/1(txdata), Modulator 4/1(txdata), Modulator 3/1(txdata), Modulator 2/1(txdata)
  Modulator 1/1(txsig) -> Merge1/1
  Modulator 2/1(txsig) -> Merge1/2
  Modulator 3/1(txsig) -> Merge1/3
  Modulator 4/1(txsig) -> Merge1/4
  Modulator 5/1(txsig) -> Merge1/5
  Modulator 6/1(txsig) -> Merge1/6
  Modulator 7/1(txsig) -> Merge1/7
  Fcn2/1 -> Modulator 1/Enable
  Fcn3/1 -> Modulator 2/Enable
  Fcn4/1 -> Modulator 3/Enable
  Fcn5/1 -> Modulator 4/Enable
  Fcn6/1 -> Modulator 5/Enable
  Fcn7/1 -> Modulator 6/Enable
  Fcn8/1 -> Modulator 7/Enable
  Fcn9/1 -> Modulator 8/Enable
  Modulator 8/1(txsig) -> Merge1/8

== system ieee80211n/ModulatorBank/Group into OFDM symbols ==
  in : Inport  Port=1  LatchInput=off
  "Group data for OFDM symbols " : simulink/Math Operations/Reshape  OutputDimensionality=Customize  OutputDimensions=[params.NSD params.OFDMSymPerFrame]
  Group into OFDM symbols : Subsystem
      mask Display: disp('Add Pilots,\nZeros')
  out : Outport
  wires:
  in/1 -> "Group data for OFDM symbols "/1
  "Group data for OFDM symbols "/1 -> Group into OFDM symbols/1(in)
  Group into OFDM symbols/1(out) -> out/1

== system ieee80211n/ModulatorBank/Group into OFDM symbols1 ==
  in : Inport  Port=1  LatchInput=off
  "Group data for OFDM symbols " : simulink/Math Operations/Reshape  OutputDimensionality=Customize  OutputDimensions=[params.NSD params.OFDMSymPerFrame]
  Group into OFDM symbols : Subsystem
      mask Display: disp('Add Pilots,\nZeros')
  out : Outport
  wires:
  in/1 -> "Group data for OFDM symbols "/1
  "Group data for OFDM symbols "/1 -> Group into OFDM symbols/1(in)
  Group into OFDM symbols/1(out) -> out/1

== system ieee80211n/ModulatorBank/Group into OFDM symbols2 ==
  in : Inport  Port=1  LatchInput=off
  "Group data for OFDM symbols " : simulink/Math Operations/Reshape  OutputDimensionality=Customize  OutputDimensions=[params.NSD params.OFDMSymPerFrame]
  Group into OFDM symbols : Subsystem
      mask Display: disp('Add Pilots,\nZeros')
  out : Outport
  wires:
  in/1 -> "Group data for OFDM symbols "/1
  "Group data for OFDM symbols "/1 -> Group into OFDM symbols/1(in)
  Group into OFDM symbols/1(out) -> out/1

== system ieee80211n/ModulatorBank/Group into OFDM symbols3 ==
  in : Inport  Port=1  LatchInput=off
  "Group data for OFDM symbols " : simulink/Math Operations/Reshape  OutputDimensionality=Customize  OutputDimensions=[params.NSD params.OFDMSymPerFrame]
  Group into OFDM symbols : Subsystem
      mask Display: disp('Add Pilots,\nZeros')
  out : Outport
  wires:
  in/1 -> "Group data for OFDM symbols "/1
  "Group data for OFDM symbols "/1 -> Group into OFDM symbols/1(in)
  Group into OFDM symbols/1(out) -> out/1
